simulink model "RTEphys"  (Simulink 8.0)
settings: Solver=VariableStepDiscrete  StartTime=0.0  StopTime=.0002  MaxStep=10e-9  RelTol=1e-3
undefined symbols (not defined in the file or in its folder): gcbh, normrnd, xlBlockLoadCallback, xlfda_numerator, xlGetNormalizedPeriod
libraries: xbsIndex_r4 x87, simulink x2, xbsEDKLib_r4 x1
(part 1 of 2)
settings Model: Creator=pdw  LastModifiedBy=pdw

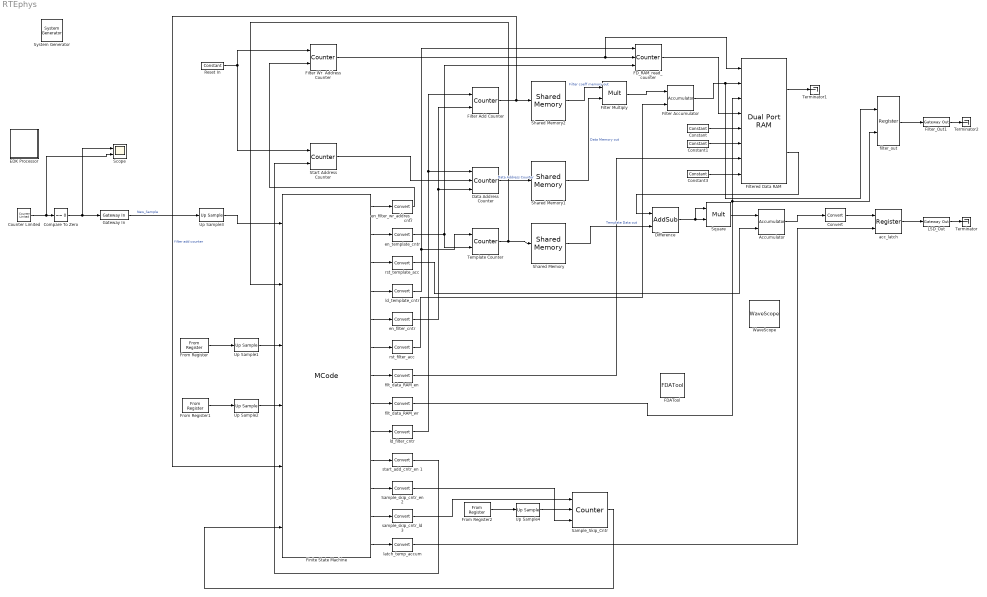
== system RTEphys ==
  " System Generator" : xbsIndex_r4/ System Generator  Tag=genX  xilinxfamily=spartan3a  part=xc3s1400an  speed=-5  package=fgg676  synthesis_tool=XST  clock_wrapper=Clock Enables  directory=./netlist  proj_type=Project Navigator  Synth_file=XST Defaults  Impl_file=ISE Defaults  testbench=off  simulink_period=.00000001  sysclk_period=10  dcm_input_clock_period=10  incr_netlist=off  trim_vbits=Everywhere in SubSystem  dbl_ovrd=According to Block Masks  core_generation=According to Block Masks  run_coregen=off  deprecated_control=off  eval_field=0  block_type=sysgen
  Accumulator : xbsIndex_r4/Accumulator  operation=Add  n_bits=24  overflow=Saturate  scale=1  rst=on  infoeditControl=reset for floating point data type must be asserted for a minimum of 2 cycles  hasbypass=off  en=off  latency=0  dbl_ovrd=off  msb_inp=100  msb=100  lsb=-100  use_behavioral_HDL=on  implementation=Fabric  block_type=accum
  Compare To Zero : simulink/Logic and Bit Operations/Compare To Zero  relop===  OutDataTypeStr=boolean  ZeroCross=off
  Constant : xbsIndex_r4/Constant  const=0  gui_display_data_type=Fixed-point  arith_type=Signed (2's comp)  n_bits=16  bin_pt=15  preci_type=Single  exp_width=8  frac_width=24  explicit_period=off  period=1  equ=P=C  opselect=C  inp2=PCIN>>17  opr=+  inp1=P  carry=CIN  dbl_ovrd=off  block_type=constant
  Constant1 : xbsIndex_r4/Constant  const=0  gui_display_data_type=Boolean  arith_type=Boolean  n_bits=16  bin_pt=14  preci_type=Single  exp_width=8  frac_width=24  explicit_period=off  period=1  equ=P=C  opselect=C  inp2=PCIN>>17  opr=+  inp1=P  carry=CIN  dbl_ovrd=off  block_type=constant
  Constant3 : xbsIndex_r4/Constant  const=1  gui_display_data_type=Boolean  arith_type=Boolean  n_bits=16  bin_pt=14  preci_type=Single  exp_width=8  frac_width=24  explicit_period=off  period=1  equ=P=C  opselect=C  inp2=PCIN>>17  opr=+  inp1=P  carry=CIN  dbl_ovrd=off  block_type=constant
  Convert : xbsIndex_r4/Convert  gui_display_data_type=Fixed-point  arith_type=Unsigned  n_bits=16  bin_pt=8  float_type=Single  exp_bits=8  fraction_bits=24  quantization=Truncate  overflow=Wrap  en=off  latency=0  dbl_ovrd=off  pipeline=off  block_type=convert
  Counter Limited : simulink/Sources/Counter Limited  uplimit=4999  tsamp=10e-9
  "Data Address Counter " : xbsIndex_r4/Counter  cnt_type=Free Running  cnt_to=Inf  operation=Down  start_count=0  cnt_by_val=1  arith_type=Unsigned  n_bits=7  bin_pt=0  load_pin=on  rst=off  en=on  explicit_period=on  period=.00000001  dbl_ovrd=off  use_behavioral_HDL=off  implementation=Fabric  block_type=counter
  Difference : xbsIndex_r4/AddSub  mode=Subtraction  use_carryin=off  use_carryout=off  en=off  latency=0  precision=User Defined  arith_type="Signed  (2's comp)"  n_bits=16  bin_pt=15  quantization=Truncate  overflow=Wrap  dbl_ovrd=off  use_behavioral_HDL=off  hw_selection=Fabric  pipelined=off  block_type=addsub
  EDK Processor : Subsystem  LoadFcn=xlBlockLoadCallback(gcbh);  mask(Xilinx EDK Processor Block){mode=EDK pcore generation, xmp=, MemVisToProc=<qt bgcolor="#FFFFFF"><div><img src="C:/Xilinx/14.7/ISE_DS/ISE/sysgen/data/images/registerplus.gif"> &lt;&lt;E1_template_size&gt;&gt;<br></div></qt>, AvailableMemories=<empty>, portInterfaceTable={'exposed'=>[],'portdir'=>[],'portname'=>[],'shortname'=>[]}, bus_type_sgadvanced=, bus_type=AXI, baseaddr=0x80000000, baseaddr_lock_sgadvanced=, baseaddr_lock=off, dual_clock_sgadvanced=, dual_clock=on, reg_readback_sgadvanced=, reg_readback=off, ucf_file=, inheritDeviceType_sgadvanced=, inheritDeviceType=off, elf_file=, codebug_sgadvanced=, codebug=on, clock_name=plb, internalPortList={}, resetPolarity=0, memxtable={'mladdr'=>[0.00000000000000000],'mlist'=>['RTEphys/From Register'],'mlname'=>['\'E1_template_size\''],'mlstate'=>[0.00000000000000000]}, procinfo={}, memmapdirty=off, blockname=, xpsintstyle=default, has_advanced_control=0, sggui_pos=-1,-1,-1,-1, block_type=edkprocessor, block_version=2.7, sg_icon_stat=62,64,-1,-1,white,blue,0,07734,right,,[ ],[ ], sg_mask_display=|, sg_list_contents={'table'=>{'AvailableMemories'=>'popup(<all>|\'E1_filter_length\'|\'E1_filter_RAM\'|\'E1_Data_RAM\'|\'E1_template_RAM\')'}}, sg_blockgui_xml=}
      mask sg_mask_display=|
      | fprintf('','COMMENT: begin icon graphics');
      | patch([0 62 62 0 0 ],[0 0 64 64 0 ],[0.77 0.82 0.91 ]);
      | plot([0 62 62 0 0 ],[0 0 64 64 0 ]);
      | patch([13.2 24.76 32.76 40.76 48.76 32.76 21.2 13.2 ],[40.88 40.88 48.88 40.88 48.88 48.88 48.88 40.88 ],[1 1 1 ]);
      | patch([21.2 32.76 24.76 13.2 21.2 ],[32.88 32.88 40.88 40.88 32.88 ],[0.931 0.946 0.973 ]);
      | patch([13.2 24.76 32.76 21.2 13.2 ],[24.88 24.88 32.88 32.88 24.88 ],[1 1 1 ]);
      | patch([21.2 48.76 40.76 32.76 24.76 13.2 21.2 ],[16.88 16.88 24.88 16.88 24.88 24.88 16.88 ],[0.931 0.946 0.973 ]);
      | fprintf('','COMMENT: end icon graphics');
      | fprintf('','COMMENT: begin icon text');
      | fprintf('','COMMENT: end icon text');
      mask prompts: mode "Configure Processor for"; xmp "XPS Project"; MemVisToProc ""; AvailableMemories "Available Memories"; portInterfaceTable ""; bus_type_sgadvanced ""; bus_type "Bus Type"; baseaddr "Base Address"; baseaddr_lock_sgadvanced ""; baseaddr_lock "Lock"; dual_clock_sgadvanced ""; dual_clock "Dual Clocks"; reg_readback_sgadvanced ""; reg_readback "Register Read-Back"; ucf_file "Constraint File"; inheritDeviceType_sgadvanced ""; inheritDeviceType "Inherit Device Type"; elf_file "Initial Program"; codebug_sgadvanced ""; codebug "Enable Co-Debug with Xilinx SDK (Beta)"; clock_name ""; internalPortList ""; resetPolarity ""; memxtable ""; procinfo ""; memmapdirty ""; blockname ""; xpsintstyle ""; has_advanced_control ""; sggui_pos ""; block_type ""; block_version ""; sg_icon_stat ""; sg_mask_display ""; sg_list_contents ""; sg_blockgui_xml ""
      mask help: Xilinx EDK Processor
      mask init:
      | try
      |   tmp_gcb = gcb;
      |   tmp_gcbh = gcbh;
      |   if (strcmp('SysGenIndex',get_param(bdroot(tmp_gcbh),'tag')) && ~isempty(regexp(bdroot(tmp_gcb), '^xbs', 'once')))
      |     return;
      |   end;
      |   xlMungeMaskParams;
      | 
      |   block_type='edkprocessor';
      | 
      |   serialized_declarations = '{''block_type''=>''String''}';
      |   xledkprocessor_init();
      |   ptable_ = xlblockprep(get_param(tmp_gcb, 'MaskWSVariables'));
      |   try
      |     xlBlockMoveCallback(tmp_gcbh);
      |   catch 
      |      clear global xl_updateicon_recursion_guard;
      |   end;
      | catch
      |   global dbgsysgen;
      |   if(~isempty(dbgsysgen) && dbgsysgen)
      |     e = regexprep(lasterr, '\n', '\nError: ');
      |     disp(['Error: While running MaskInit code on block ' tmp_gcb ': ' e]);
      |     error(e);
      |   end
      | end
      settings: CopyFcn=xlProcBlockCopyCallback(gcbh);xlBlockMoveCallback(gcbh);  DeleteFcn=xlDestroyGui(gcbh);  ModelCloseFcn=xlDestroyGui(gcbh);  PreSaveFcn=xlBlockPreSaveCallback(gcbh);  PostSaveFcn=xlBlockPostSaveCallback(gcbh);  DestroyFcn=xlDestroyGui(gcbh);  OpenFcn=bh=gcbh;xlProcBlockCallbacks('populatesharedmemorylistbox',bh);xlOpenGui(bh, 'edkprocessor_gui.xml', @xlProcBlockEnablement, @xlProcBlockAction);  CloseFcn=xlDestroyGui(gcbh);  MoveFcn=xlBlockMoveCallback(gcbh);
      mask Help: eval('');xlDoc('-book','sysgen','-topic','EDK_Processor');
      mask TypeOptions mode: EDK pcore generation | HDL netlisting
      mask TypeOptions bus_type: AXI | PLB
      mask Display:
      | fprintf('','COMMENT: begin icon graphics');
      | patch([0 62 62 0 0 ],[0 0 64 64 0 ],[0.77 0.82 0.91 ]);
      | plot([0 62 62 0 0 ],[0 0 64 64 0 ]);
      | patch([13.2 24.76 32.76 40.76 48.76 32.76 21.2 13.2 ],[40.88 40.88 48.88 40.88 48.88 48.88 48.88 40.88 ],[1 1 1 ]);
      | patch([21.2 32.76 24.76 13.2 21.2 ],[32.88 32.88 40.88 40.88 32.88 ],[0.931 0.946 0.973 ]);
      | patch([13.2 24.76 32.76 21.2 13.2 ],[24.88 24.88 32.88 32.88 24.88 ],[1 1 1 ]);
      | patch([21.2 48.76 40.76 32.76 24.76 13.2 21.2 ],[16.88 16.88 24.88 16.88 24.88 24.88 16.88 ],[0.931 0.946 0.973 ]);
      | fprintf('','COMMENT: end icon graphics');
      | fprintf('','COMMENT: begin icon text');
      | disp('');
      | 
      | fprintf('','COMMENT: end icon text');
  FDATool : xbsIndex_r4/FDATool  block_type=fdatool
      settings: infoedit=FDATool
  FD_RAM_read_counter : xbsIndex_r4/Counter  cnt_type=Free Running  cnt_to=Inf  operation=Down  start_count=0  cnt_by_val=1  arith_type=Unsigned  n_bits=7  bin_pt=0  load_pin=on  rst=off  en=on  explicit_period=on  period=.00000001  dbl_ovrd=off  use_behavioral_HDL=off  implementation=Fabric  block_type=counter
  "Filter Accumulator " : xbsIndex_r4/Accumulator  operation=Add  n_bits=16  overflow=Wrap  scale=1  rst=on  infoeditControl=reset for floating point data type must be asserted for a minimum of 2 cycles  hasbypass=off  en=off  latency=0  dbl_ovrd=off  msb_inp=100  msb=100  lsb=-100  use_behavioral_HDL=on  implementation=Fabric  block_type=accum
  Filter Add Counter : xbsIndex_r4/Counter  cnt_type=Free Running  cnt_to=Inf  operation=Up  start_count=0  cnt_by_val=1  arith_type=Unsigned  n_bits=7  bin_pt=0  load_pin=off  rst=on  en=on  explicit_period=on  period=.00000001  dbl_ovrd=off  use_behavioral_HDL=off  implementation=Fabric  block_type=counter
  Filter Multiply : xbsIndex_r4/Mult  precision=User Defined  arith_type="Signed  (2's comp)"  n_bits=16  bin_pt=15  quantization=Truncate  overflow=Wrap  en=off  latency=3  dbl_ovrd=off  use_behavioral_HDL=off  opt=Speed  use_embedded=on  optimum_pipeline=on  pipeline=on  use_rpm=on  placement_style=Triangular  block_type=mult
  Filter Wr  Address Counter : xbsIndex_r4/Counter  cnt_type=Free Running  cnt_to=Inf  operation=Up  start_count=0  cnt_by_val=1  arith_type=Unsigned  n_bits=7  bin_pt=0  load_pin=off  rst=on  en=on  explicit_period=off  period=.00005  dbl_ovrd=off  use_behavioral_HDL=off  implementation=Fabric  block_type=counter
  Filter_Out1 : xbsIndex_r4/Gateway Out  inherit_from_input=off  hdl_port=on  timing_constraint=None  locs_specified=off  LOCs={}  UseAsDAC=off  DACChannel='1'  block_type=gatewayout
  Filtered Data RAM : xbsIndex_r4/Dual Port RAM  depth=128  initVector=[0.1*ones(1,128)]  distributed_mem=Block RAM  init_a=0  init_b=0  rst_a=off  rst_b=off  en_a=on  en_b=on  latency=1  write_mode_A=Read After Write  write_mode_B=Read After Write  dbl_ovrd=off  optimize=Area  block_type=dpram
  Finite State Machine : xbsIndex_r4/MCode  mfname=cnt_state_machine  explicit_period=off  period=1  inputsTable={'boundInpExpr'=>['','','','','','',''],'inputs'=>['new_sample_available','template_cnt','template_size','filter_length','filter_cntr','samples_to_skip','sample_skip_cntr']}  outputsTable={'outputs'=>['en_filter_wr_address_cntr','en_template_cntr','rst_template_acc','ld_template_cntr','en_filter_cntr','rst_filter_acc','filt_data_RAM_en','filt_data_RAM_wr','ld_filter_cntr','start_add_cntr_en','sample_skip_cntr_en','sample_skip_cntr_ld'],'suppressOut'=>['off','off','off','off','off','off','off','off','off','off','off','off']}  dbl_ovrd=off  enable_stdout=off  enable_debug=off  suppress_output=on  defparams={}  hide_port_list={}  block_type=mcode
  From Register : xbsIndex_r4/From Register  shared_memory_name='E1_template_size'  init=50  period=1  ownership=Locally owned and initialized  gui_display_data_type=Fixed-point  arith_type=Unsigned  n_bits=16  bin_pt=0  preci_type=Single  dbl_ovrd=off  block_type=fromreg
      settings: AttributesFormatString=<< %<shared_memory_name> >>  infoedit="Register block that reads data to a shared memory register.  Delay of one sample period."
  From Register1 : xbsIndex_r4/From Register  shared_memory_name='E1_filter_length'  init=48  period=1  ownership=Locally owned and initialized  gui_display_data_type=Fixed-point  arith_type=Unsigned  n_bits=16  bin_pt=0  preci_type=Single  dbl_ovrd=off  block_type=fromreg
      settings: AttributesFormatString=<< %<shared_memory_name> >>  infoedit="Register block that reads data to a shared memory register.  Delay of one sample period."
  From Register2 : xbsIndex_r4/From Register  shared_memory_name='E1_samples_to_skip'  init=0  period=1  ownership=Locally owned and initialized  gui_display_data_type=Fixed-point  arith_type=Unsigned  n_bits=8  bin_pt=0  preci_type=Single  dbl_ovrd=off  block_type=fromreg
      settings: AttributesFormatString=<< %<shared_memory_name> >>  infoedit="Register block that reads data to a shared memory register.  Delay of one sample period."
  Gateway In : xbsIndex_r4/Gateway In  gui_display_data_type=Boolean  arith_type=Boolean  n_bits=16  bin_pt=14  preci_type=Single  exp_width=8  frac_width=24  quantization="Round  (unbiased: +/- Inf)"  overflow=Saturate  period=1  dbl_ovrd=off  timing_constraint=Data Rate  locs_specified=off  LOCs={}  UseAsADC=off  ADCChannel='1'  inherit_from_input=off  hdl_port=on  block_type=gatewayin
  LSD_Out : xbsIndex_r4/Gateway Out  inherit_from_input=off  hdl_port=on  timing_constraint=None  locs_specified=off  LOCs={}  UseAsDAC=off  DACChannel='1'  block_type=gatewayout
  Reset In : xbsIndex_r4/Constant  const=0  gui_display_data_type=Boolean  arith_type=Boolean  n_bits=16  bin_pt=14  preci_type=Single  exp_width=8  frac_width=24  explicit_period=off  period=1  equ=P=C  opselect=C  inp2=PCIN>>17  opr=+  inp1=P  carry=CIN  dbl_ovrd=off  block_type=constant
  "Sample_Skip_Cntr " : xbsIndex_r4/Counter  cnt_type=Free Running  cnt_to=Inf  operation=Down  start_count=0  cnt_by_val=1  arith_type=Unsigned  n_bits=8  bin_pt=0  load_pin=on  rst=off  en=on  explicit_period=on  period=.00000001  dbl_ovrd=off  use_behavioral_HDL=off  implementation=Fabric  block_type=counter
  Sample_skip_cntr_en 2 : xbsIndex_r4/Convert  gui_display_data_type=Boolean  arith_type=Boolean  n_bits=16  bin_pt=14  float_type=Single  exp_bits=8  fraction_bits=24  quantization=Truncate  overflow=Wrap  en=off  latency=0  dbl_ovrd=off  pipeline=off  block_type=convert
  Scope : Scope  NumInputPorts=2
      settings: YMin=-5~-5  YMax=5~5  MaxDataPoints=510000
  Shared Memory : xbsIndex_r4/Shared Memory  shared_memory_name='E1_template_RAM'  depth=128  ownership=Locally Owned and Initialized  initVector=fliplr(0.8*sin(2*pi*(0:49)/50))  en=off  mutex=Unprotected  mode=Read Only  write_mode=Read After Write  time_out=0  latency=1  explicit_data_type=on  gui_display_data_type=Fixed-point  arith_type="Signed  (2's comp)"  n_bits=16  bin_pt=15  preci_type=Single  implementation=Block RAM  use_rpm=off  block_type=shmem
      settings: AttributesFormatString=<< %<shared_memory_name> >>
  Shared Memory1 : xbsIndex_r4/Shared Memory  shared_memory_name='E1_Data_RAM'  depth=128  ownership=Locally Owned and Initialized  initVector="([0*(1:32) 0.8*sin(2*pi*(0:49)/50) 0*(1:46)  ] + 0.1 + normrnd(0, .01, [1,128]))"  en=off  mutex=Unprotected  mode=Read Only  write_mode=Read After Write  time_out=0  latency=1  explicit_data_type=on  gui_display_data_type=Fixed-point  arith_type="Signed  (2's comp)"  n_bits=16  bin_pt=15  preci_type=Single  implementation=Block RAM  use_rpm=off  block_type=shmem
      settings: AttributesFormatString=<< %<shared_memory_name> >>
  Shared Memory2 : xbsIndex_r4/Shared Memory  shared_memory_name='E1_filter_RAM'  depth=128  ownership=Locally Owned and Initialized  initVector=xlfda_numerator ('FDATool')  en=off  mutex=Unprotected  mode=Read Only  write_mode=Read After Write  time_out=0  latency=1  explicit_data_type=on  gui_display_data_type=Fixed-point  arith_type="Signed  (2's comp)"  n_bits=16  bin_pt=15  preci_type=Single  implementation=Block RAM  use_rpm=off  block_type=shmem
      settings: AttributesFormatString=<< %<shared_memory_name> >>
  Square : xbsIndex_r4/Mult  precision=User Defined  arith_type=Unsigned  n_bits=16  bin_pt=15  quantization=Truncate  overflow=Saturate  en=off  latency=3  dbl_ovrd=off  use_behavioral_HDL=off  opt=Speed  use_embedded=on  optimum_pipeline=off  pipeline=on  use_rpm=on  placement_style=Triangular  block_type=mult
  Start Address Counter : xbsIndex_r4/Counter  cnt_type=Free Running  cnt_to=Inf  operation=Up  start_count=0  cnt_by_val=1  arith_type=Unsigned  n_bits=7  bin_pt=0  load_pin=off  rst=on  en=on  explicit_period=off  period=.00005  dbl_ovrd=off  use_behavioral_HDL=off  implementation=Fabric  block_type=counter
  Template Counter : xbsIndex_r4/Counter  cnt_type=Free Running  cnt_to=Inf  operation=Up  start_count=0  cnt_by_val=1  arith_type=Unsigned  n_bits=7  bin_pt=0  load_pin=off  rst=on  en=on  explicit_period=on  period=.00000001  dbl_ovrd=off  use_behavioral_HDL=off  implementation=Fabric  block_type=counter
  Terminator : Terminator
  Terminator1 : Terminator
  Terminator2 : Terminator
  Up Sample{1..4} (4 alike) : xbsIndex_r4/Up Sample  sample_ratio=10^8  copy_samples=on  en=off  latency=0  dbl_ovrd=off  block_type=usamp
  WaveScope : xbsIndex_r4/WaveScope  block_type=wavescope
  "acc_latch " : xbsIndex_r4/Register  init=0  rst=off  en=on  dbl_ovrd=off  block_type=register
  en_filter_cntr : xbsIndex_r4/Convert  gui_display_data_type=Boolean  arith_type=Boolean  n_bits=16  bin_pt=14  float_type=Single  exp_bits=8  fraction_bits=24  quantization=Truncate  overflow=Wrap  en=off  latency=0  dbl_ovrd=off  pipeline=off  block_type=convert
  en_filter_wr_addres_cntr : xbsIndex_r4/Convert  gui_display_data_type=Boolean  arith_type=Boolean  n_bits=16  bin_pt=14  float_type=Single  exp_bits=8  fraction_bits=24  quantization=Truncate  overflow=Wrap  en=off  latency=0  dbl_ovrd=off  pipeline=off  block_type=convert
  en_template_cntr : xbsIndex_r4/Convert  gui_display_data_type=Boolean  arith_type=Boolean  n_bits=16  bin_pt=14  float_type=Single  exp_bits=8  fraction_bits=24  quantization=Truncate  overflow=Wrap  en=off  latency=0  dbl_ovrd=off  pipeline=off  block_type=convert
  filt_data_RAM_en : xbsIndex_r4/Convert  gui_display_data_type=Boolean  arith_type=Boolean  n_bits=16  bin_pt=14  float_type=Single  exp_bits=8  fraction_bits=24  quantization=Truncate  overflow=Wrap  en=off  latency=0  dbl_ovrd=off  pipeline=off  block_type=convert
  filt_data_RAM_wr : xbsIndex_r4/Convert  gui_display_data_type=Boolean  arith_type=Boolean  n_bits=16  bin_pt=14  float_type=Single  exp_bits=8  fraction_bits=24  quantization=Truncate  overflow=Wrap  en=off  latency=0  dbl_ovrd=off  pipeline=off  block_type=convert
  filter_out : xbsIndex_r4/Register  init=0  rst=off  en=on  dbl_ovrd=off  block_type=register
  latch_temp_accum : xbsIndex_r4/Convert  gui_display_data_type=Boolean  arith_type=Boolean  n_bits=16  bin_pt=14  float_type=Single  exp_bits=8  fraction_bits=24  quantization=Truncate  overflow=Wrap  en=off  latency=0  dbl_ovrd=off  pipeline=off  block_type=convert
  "ld_filter_cntr " : xbsIndex_r4/Convert  gui_display_data_type=Boolean  arith_type=Boolean  n_bits=16  bin_pt=14  float_type=Single  exp_bits=8  fraction_bits=24  quantization=Truncate  overflow=Wrap  en=off  latency=0  dbl_ovrd=off  pipeline=off  block_type=convert
  ld_template_cntr : xbsIndex_r4/Convert  gui_display_data_type=Boolean  arith_type=Boolean  n_bits=16  bin_pt=14  float_type=Single  exp_bits=8  fraction_bits=24  quantization=Truncate  overflow=Wrap  en=off  latency=0  dbl_ovrd=off  pipeline=off  block_type=convert
  rst_filter_acc : xbsIndex_r4/Convert  gui_display_data_type=Boolean  arith_type=Boolean  n_bits=16  bin_pt=14  float_type=Single  exp_bits=8  fraction_bits=24  quantization=Truncate  overflow=Wrap  en=off  latency=0  dbl_ovrd=off  pipeline=off  block_type=convert
  rst_template_acc : xbsIndex_r4/Convert  gui_display_data_type=Boolean  arith_type=Boolean  n_bits=16  bin_pt=14  float_type=Single  exp_bits=8  fraction_bits=24  quantization=Truncate  overflow=Wrap  en=off  latency=0  dbl_ovrd=off  pipeline=off  block_type=convert
  sample_skip_cntr_ld 3 : xbsIndex_r4/Convert  gui_display_data_type=Boolean  arith_type=Boolean  n_bits=16  bin_pt=14  float_type=Single  exp_bits=8  fraction_bits=24  quantization=Truncate  overflow=Wrap  en=off  latency=0  dbl_ovrd=off  pipeline=off  block_type=convert
  start_add_cntr_en 1 : xbsIndex_r4/Convert  gui_display_data_type=Boolean  arith_type=Boolean  n_bits=16  bin_pt=14  float_type=Single  exp_bits=8  fraction_bits=24  quantization=Truncate  overflow=Wrap  en=off  latency=0  dbl_ovrd=off  pipeline=off  block_type=convert
  wires:
  Start Address Counter/1 -> "Data Address Counter "/2
  Template Counter/1 -> Finite State Machine/2, Shared Memory/1
  Square/1 -> Accumulator/1
  ld_template_cntr/1 -> FD_RAM_read_counter/1, Template Counter/1
  From Register/1 -> Up Sample1/1
  "Data Address Counter "/1 -> Shared Memory1/1  "Data Address Counter"
  en_template_cntr/1 -> Template Counter/2, FD_RAM_read_counter/3
  rst_template_acc/1 -> Accumulator/2
  Difference/1 -> Square/1, Square/2
  Up Sample1/1 -> Finite State Machine/3
  Filter Add Counter/1 -> Finite State Machine/5, Shared Memory2/1  "filter add counter"
  Shared Memory1/1 -> Filter Multiply/2  "Data Memory out"
  Shared Memory2/1 -> Filter Multiply/1  "Filter coeff memory out"
  Filter Multiply/1 -> "Filter Accumulator "/1
  From Register1/1 -> Up Sample2/1
  Up Sample2/1 -> Finite State Machine/4
  rst_filter_acc/1 -> "Filter Accumulator "/2
  "Filter Accumulator "/1 -> filter_out/1, Filtered Data RAM/2
  Constant/1 -> Filtered Data RAM/5
  Constant1/1 -> Filtered Data RAM/6
  filt_data_RAM_wr/1 -> filter_out/2, Filtered Data RAM/3
  en_filter_cntr/1 -> "Data Address Counter "/3, Filter Add Counter/2
  filt_data_RAM_en/1 -> Filtered Data RAM/7
  "ld_filter_cntr "/1 -> "Data Address Counter "/1, Filter Add Counter/1
  Accumulator/1 -> Convert/1
  FD_RAM_read_counter/1 -> Filtered Data RAM/4
  start_add_cntr_en 1/1 -> Start Address Counter/2
  Gateway In/1 -> Up Sample3/1  "New_Sample"
  Counter Limited/1 -> Scope/2, Compare To Zero/1
  Compare To Zero/1 -> Scope/1, Gateway In/1
  Up Sample3/1 -> Finite State Machine/1
  Filter Wr  Address Counter/1 -> Filtered Data RAM/1, FD_RAM_read_counter/2
  From Register2/1 -> Up Sample4/1
  Up Sample4/1 -> "Sample_Skip_Cntr "/2
  Finite State Machine/11 -> Sample_skip_cntr_en 2/1
  Finite State Machine/12 -> sample_skip_cntr_ld 3/1
  sample_skip_cntr_ld 3/1 -> "Sample_Skip_Cntr "/1
  Sample_skip_cntr_en 2/1 -> "Sample_Skip_Cntr "/3
  Finite State Machine/10 -> start_add_cntr_en 1/1
  Finite State Machine/9 -> "ld_filter_cntr "/1
  Finite State Machine/8 -> filt_data_RAM_wr/1
  Finite State Machine/7 -> filt_data_RAM_en/1
  Finite State Machine/6 -> rst_filter_acc/1
  Finite State Machine/5 -> en_filter_cntr/1
  Finite State Machine/4 -> ld_template_cntr/1
  Finite State Machine/3 -> rst_template_acc/1
  Finite State Machine/2 -> en_template_cntr/1
  Finite State Machine/1 -> en_filter_wr_addres_cntr/1
  en_filter_wr_addres_cntr/1 -> Filter Wr  Address Counter/2
  Filtered Data RAM/2 -> Difference/1
  Reset In/1 -> Start Address Counter/1, Filter Wr  Address Counter/1
  "Sample_Skip_Cntr "/1 -> Finite State Machine/6
  "acc_latch "/1 -> LSD_Out/1
  LSD_Out/1 -> Terminator/1
  Constant3/1 -> Filtered Data RAM/8
  Filtered Data RAM/1 -> Terminator1/1
  Shared Memory/1 -> Difference/2  "Template Data out"
  Finite State Machine/13 -> latch_temp_accum/1
  latch_temp_accum/1 -> "acc_latch "/2
  Convert/1 -> "acc_latch "/1
  Filter_Out1/1 -> Terminator2/1
  filter_out/1 -> Filter_Out1/1
